simulink model "test_model"  (R2016b)
settings: Solver=ode23tb  StartTime=0.0  StopTime=500  RelTol=1e-3
libraries: AERO x1, ATM x1, EOM x1, MASS x1, MOT_lib x1
settings Model: Creator=Andrew  LastModifiedBy=Andrew
settings DataIOCC: SaveState=on

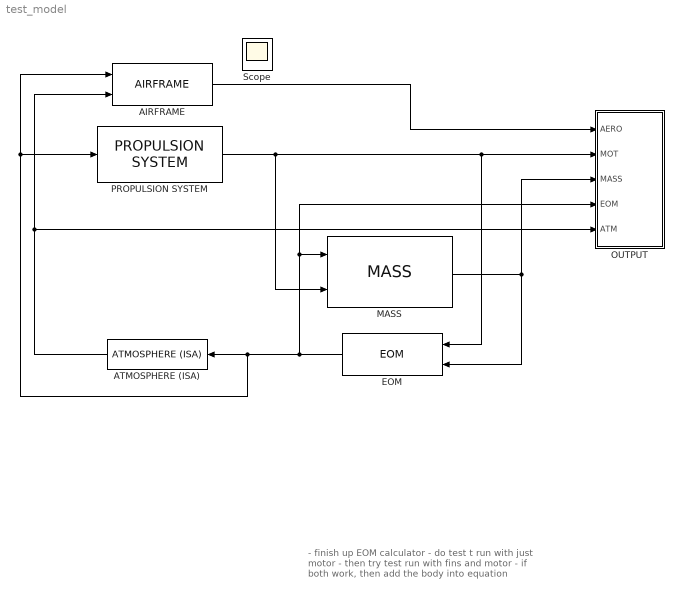
== system test_model ==
  note: - finish up EOM calculator
      | - do test t run with just motor
      | - then try test run with fins and motor
      | - if both work, then add the body into equation
  AIRFRAME : AERO/AIRFRAME
  ATMOSPHERE (ISA) : ATM/ATMOSPHERE (ISA)
  EOM : EOM/EOM
  MASS : MASS/MASS
  OUTPUT : Subsystem
  PROPULSION SYSTEM : MOT_lib/PROPULSION SYSTEM
  Scope : Scope
  wires:
  PROPULSION SYSTEM/1 -> MASS/2, EOM/1, OUTPUT/2(MOT)
  MASS/1 -> EOM/2, OUTPUT/3(MASS)
  EOM/1 -> AIRFRAME/1, PROPULSION SYSTEM/1, ATMOSPHERE (ISA)/1, MASS/1, OUTPUT/4(EOM)
  ATMOSPHERE (ISA)/1 -> AIRFRAME/2, OUTPUT/5(ATM)
  AIRFRAME/1 -> OUTPUT/1(AERO)

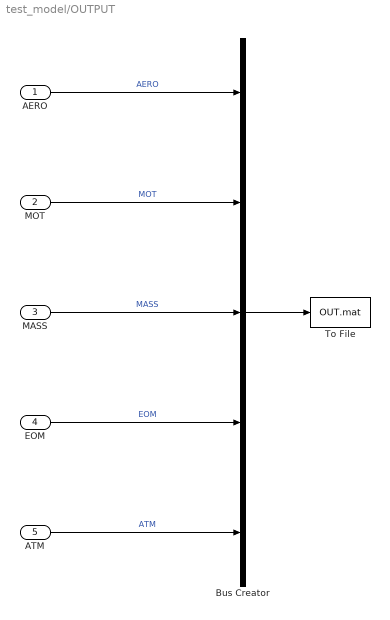
== system test_model/OUTPUT ==
  AERO : Inport
  MOT : Inport  Port=2
  MASS : Inport  Port=3
  EOM : Inport  Port=4
  ATM : Inport  Port=5
  Bus Creator : BusCreator  Inputs=5
  To File : ToFile  Filename=OUT.mat  MatrixName=OUT  SaveFormat=Timeseries
  wires:
  Bus Creator/1 -> To File/1
  AERO/1 -> Bus Creator/1  "AERO"
  ATM/1 -> Bus Creator/5  "ATM"
  EOM/1 -> Bus Creator/4  "EOM"
  MASS/1 -> Bus Creator/3  "MASS"
  MOT/1 -> Bus Creator/2  "MOT"
